simulink model "Admittace_Control"  (R2020a)
settings: Solver=FixedStepAuto  StartTime=0.0  StopTime=2  FixedStep=0.001  RelTol=1e-3  EnableMultiTasking=on
undefined symbols (not defined in the file or in its folder): X, Y, Z
libraries: sm_lib x79, nesl_utility x41, roblocks x8
(part 1 of 3)
settings Model: Creator=Administrator  LastModifiedBy=hemingshan
settings DataIOCC: ReturnWorkspaceOutputs=off
settings OptimizationCC: LifeSpan=inf
settings DebuggingCC: SFUnexpectedBacktrackingDiag=warning  SFNoUnconditionalDefaultTransitionDiag=warning  ArithmeticOperatorsInVariantConditions=warning
settings SFSimCC: SimUseLocalCustomCode=off  CustomCodeUndefinedFunction=UseInterfaceOnly
settings RTWCC: RTWUseLocalCustomCode=off
settings CodeAppCC: StateflowObjectComments=on
settings GRTTargetCC: TargetLangStandard=C89/C90 (ANSI)
settings ConfigComp: CovMetricSettings=dw  CovHtmlReporting=on  CovSaveCumulativeToWorkspaceVar=on  CovSaveSingleToWorkspaceVar=on  CovExternalEMLEnable=off
settings SimscapeCC: SimscapeNormalizeSystem=off

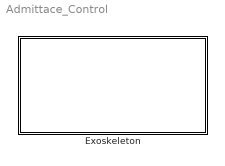
== system Admittace_Control ==
  Exoskeleton : Subsystem
      mask Display: disp('Admittance Control');

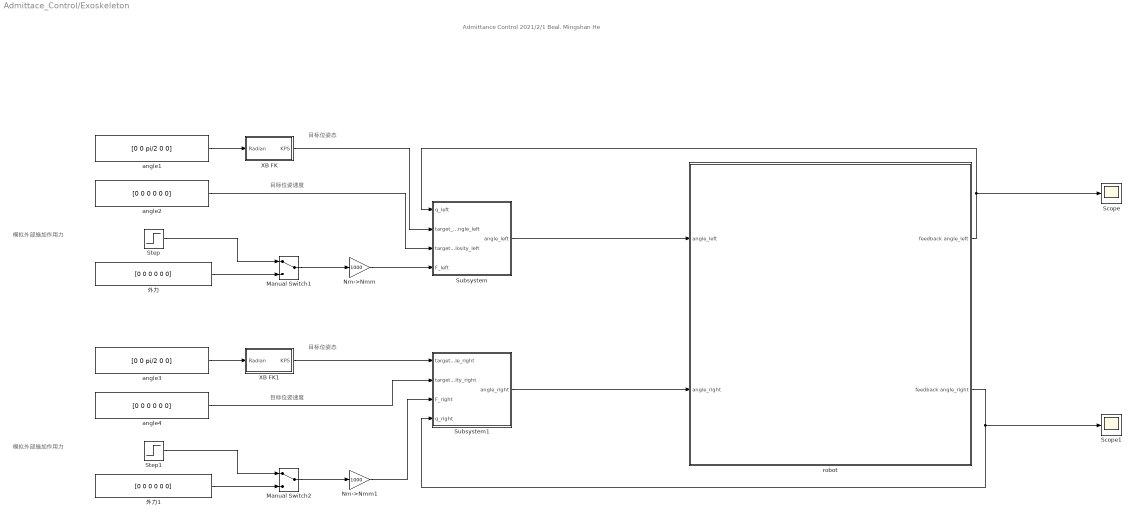
== system Admittace_Control/Exoskeleton ==
  note: Admittance Control
      | 2021/2/1
      | Beal. Mingshan He
  note: 目标位姿速度
  note: 目标位姿态
  note: 模拟外部施加作用力
  note: 模拟外部施加作用力
  note: 目标位姿速度
  note: 目标位姿态
  Manual Switch1 : ManualSwitch
  Manual Switch2 : ManualSwitch
  Nm->Nmm : Gain  Gain=1000
  Nm->Nmm1 : Gain  Gain=1000
  Scope : Scope
  Scope1 : Scope
  Step : Step  Before=[0.1 0 10 0 0 0]  After=[0 0 0 0 0 0]  SampleTime=0
  Step1 : Step  Before=[0.1 0 10 0 0 0]  After=[0 0 0 0 0 0]  SampleTime=0
  Subsystem : Subsystem
  Subsystem1 : Subsystem
  XB FK : Subsystem
  XB FK1 : Subsystem
  angle1 : Constant  Value=[0 0 pi/2 0 0]
  angle2 : Constant  Value=[0 0 0 0 0 0]
  angle3 : Constant  Value=[0 0 pi/2 0 0]
  angle4 : Constant  Value=[0 0 0 0 0 0]
  robot : Subsystem
  外力 : Constant  Value=[0 0 0 0 0 0]
  外力1 : Constant  Value=[0 0 0 0 0 0]
  wires:
  Step/1 -> Manual Switch1/1
  angle1/1 -> XB FK/1(Radian)
  Manual Switch1/1 -> Nm->Nmm/1
  外力/1 -> Manual Switch1/2
  robot/1(feedback angle_left) -> Subsystem/1(q_left), Scope/1
  XB FK/1(KPS) -> Subsystem/2(target_angle_left)
  angle2/1 -> Subsystem/3(target_velosity_left)
  Nm->Nmm/1 -> Subsystem/4(F_left)
  Subsystem/1(angle_left) -> robot/1(angle_left)
  Subsystem1/1(angle_right) -> robot/2(angle_right)
  robot/2(feedback angle_right) -> Subsystem1/4(q_right), Scope1/1
  Nm->Nmm1/1 -> Subsystem1/3(F_right)
  Manual Switch2/1 -> Nm->Nmm1/1
  Step1/1 -> Manual Switch2/1
  外力1/1 -> Manual Switch2/2
  angle3/1 -> XB FK1/1(Radian)
  XB FK1/1(KPS) -> Subsystem1/1(target_angle_right)
  angle4/1 -> Subsystem1/2(target_velosity_right)

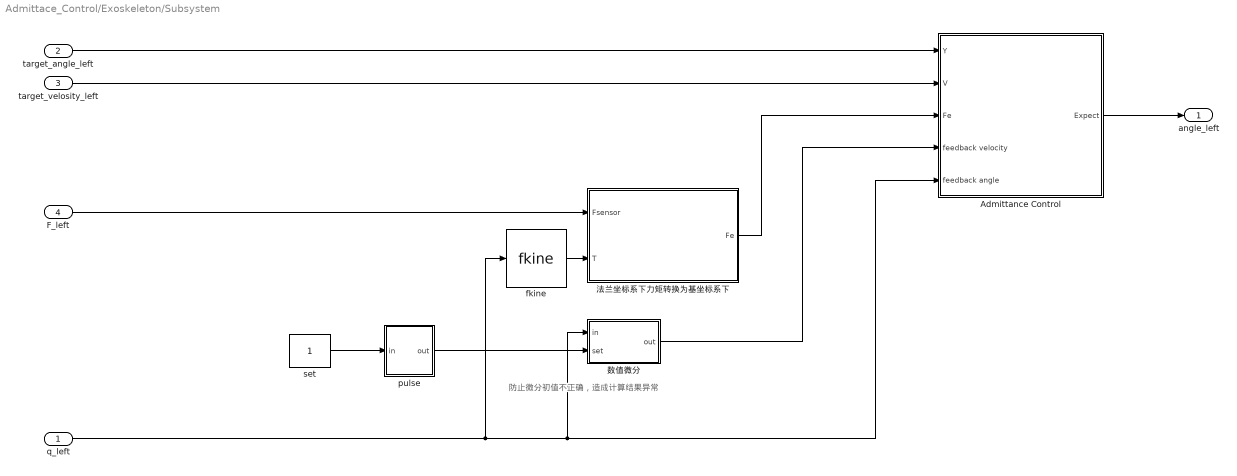
== system Admittace_Control/Exoskeleton/Subsystem ==
  note: 防止微分初值不正确，造成计算结果异常
  q_left : Inport
  target_angle_left : Inport  Port=2
  target_velosity_left : Inport  Port=3
  F_left : Inport  Port=4
  Admittance Control : Subsystem  mask{m_M=[1 1 1 1 1 1], m_B=[100 100 100 200 200 200], m_K=[250 250 250 1000 1000 1000]}
      mask prompts: m_M "M"; m_B "B"; m_K "K"
  fkine : roblocks/Arm/fkine  robot=robot
  pulse : MATLAB Function  TreatAsAtomicUnit=on
  set : Constant
  数值微分 : MATLAB Function  TreatAsAtomicUnit=on
  法兰坐标系下力矩转换为基坐标系下 : MATLAB Function  TreatAsAtomicUnit=on
  angle_left : Outport
  wires:
  fkine/1 -> 法兰坐标系下力矩转换为基坐标系下/2(T)
  法兰坐标系下力矩转换为基坐标系下/1(Fe) -> Admittance Control/3(Fe)
  pulse/1(out) -> 数值微分/2(set)
  target_angle_left/1 -> Admittance Control/1(Y)
  数值微分/1(out) -> Admittance Control/4(feedback velocity)
  F_left/1 -> 法兰坐标系下力矩转换为基坐标系下/1(Fsensor)
  set/1 -> pulse/1(in)
  q_left/1 -> Admittance Control/5(feedback angle), 数值微分/1(in), fkine/1
  target_velosity_left/1 -> Admittance Control/2(V)
  Admittance Control/1(Expect) -> angle_left/1

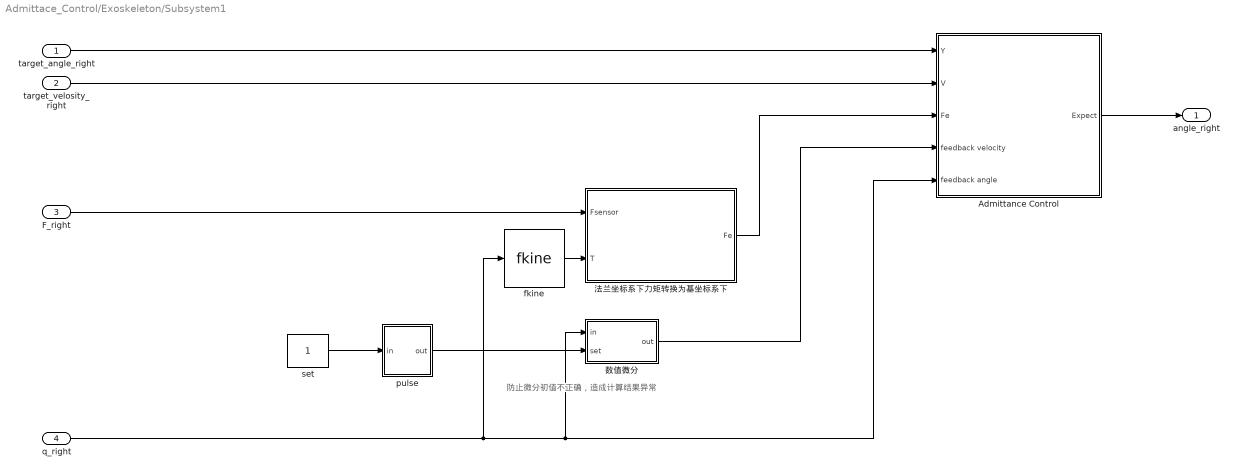
== system Admittace_Control/Exoskeleton/Subsystem1 ==
  note: 防止微分初值不正确，造成计算结果异常
  target_angle_right : Inport
  target_velosity_right : Inport  Port=2
  F_right : Inport  Port=3
  q_right : Inport  Port=4
  Admittance Control : Subsystem  mask{m_M=[1 1 1 1 1 1], m_B=[100 100 100 200 200 200], m_K=[250 250 250 1000 1000 1000]}
      mask prompts: m_M "M"; m_B "B"; m_K "K"
  fkine : roblocks/Arm/fkine  robot=robot
  pulse : MATLAB Function  TreatAsAtomicUnit=on
  set : Constant
  数值微分 : MATLAB Function  TreatAsAtomicUnit=on
  法兰坐标系下力矩转换为基坐标系下 : MATLAB Function  TreatAsAtomicUnit=on
  angle_right : Outport
  wires:
  fkine/1 -> 法兰坐标系下力矩转换为基坐标系下/2(T)
  法兰坐标系下力矩转换为基坐标系下/1(Fe) -> Admittance Control/3(Fe)
  pulse/1(out) -> 数值微分/2(set)
  target_angle_right/1 -> Admittance Control/1(Y)
  数值微分/1(out) -> Admittance Control/4(feedback velocity)
  F_right/1 -> 法兰坐标系下力矩转换为基坐标系下/1(Fsensor)
  set/1 -> pulse/1(in)
  q_right/1 -> Admittance Control/5(feedback angle), 数值微分/1(in), fkine/1
  target_velosity_right/1 -> Admittance Control/2(V)
  Admittance Control/1(Expect) -> angle_right/1

== system Admittace_Control/Exoskeleton/XB FK ==
  Radian : Inport
  DH-CC1 : MATLAB Function  TreatAsAtomicUnit=on
  fkine1 : roblocks/Arm/fkine  robot=robot
  KPS : Outport  VectorParamsAs1DForOutWhenUnconnected=off
  wires:
  fkine1/1 -> DH-CC1/1(KPS44)
  DH-CC1/1(KPS6) -> KPS/1
  Radian/1 -> fkine1/1

== system Admittace_Control/Exoskeleton/XB FK1 ==
  Radian : Inport
  DH-CC1 : MATLAB Function  TreatAsAtomicUnit=on
  fkine1 : roblocks/Arm/fkine  robot=robot
  KPS : Outport  VectorParamsAs1DForOutWhenUnconnected=off
  wires:
  fkine1/1 -> DH-CC1/1(KPS44)
  DH-CC1/1(KPS6) -> KPS/1
  Radian/1 -> fkine1/1

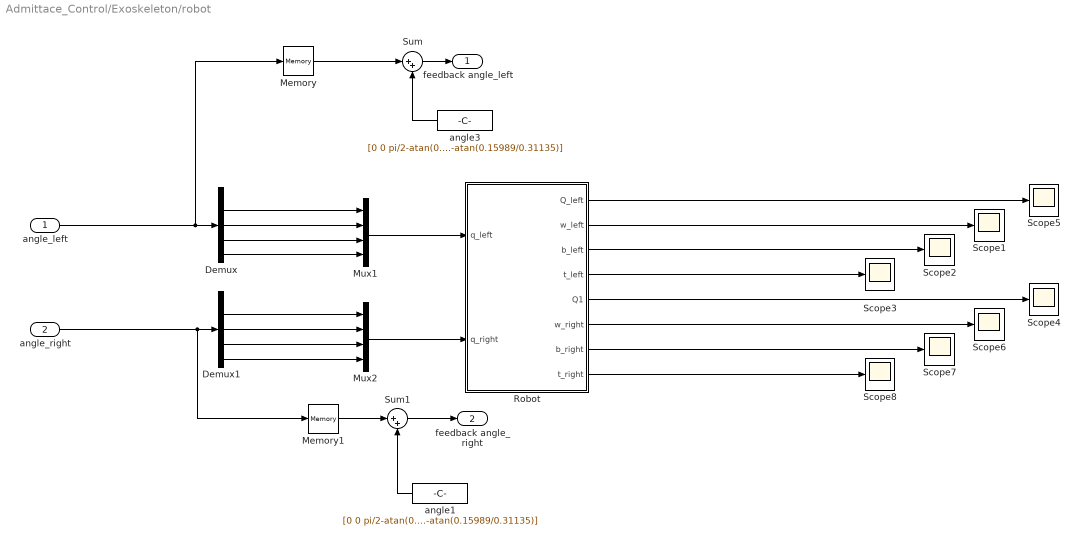
== system Admittace_Control/Exoskeleton/robot ==
  angle_left : Inport
  angle_right : Inport  Port=2
  Demux : Demux  Outputs=5
  Demux1 : Demux  Outputs=5
  Memory : Memory  InitialCondition=[0 0 0 0 0]
  Memory1 : Memory  InitialCondition=[0 0 0 0 0]
  Mux1 : Mux
  Mux2 : Mux
  Robot : Subsystem
  Scope{1..8} (8 alike) : Scope
  Sum : Sum  Inputs=|++
  Sum1 : Sum  Inputs=|++
  angle1 : Constant  Value=[0 0 pi/2-atan(0.23966/0.28189) pi/2-atan(0.23966/0.28189)+atan(0.15989/0.31135) -atan(0.15989/0.31135)]
  angle3 : Constant  Value=[0 0 pi/2-atan(0.23966/0.28189) pi/2-atan(0.23966/0.28189)+atan(0.15989/0.31135) -atan(0.15989/0.31135)]
  feedback angle_left : Outport  VectorParamsAs1DForOutWhenUnconnected=off
  feedback angle_right : Outport  Port=2  VectorParamsAs1DForOutWhenUnconnected=off
  wires:
  Robot/1(Q_left) -> Scope5/1
  Robot/2(w_left) -> Scope1/1
  Robot/3(b_left) -> Scope2/1
  Robot/4(t_left) -> Scope3/1
  angle_left/1 -> Memory/1, Demux/1
  Mux1/1 -> Robot/1(q_left)
  Demux/2 -> Mux1/1
  Demux/3 -> Mux1/2
  Demux/4 -> Mux1/3
  Demux/5 -> Mux1/4
  Robot/5(Q1) -> Scope4/1
  Robot/6(w_right) -> Scope6/1
  Robot/7(b_right) -> Scope7/1
  Robot/8(t_right) -> Scope8/1
  angle_right/1 -> Memory1/1, Demux1/1
  Demux1/5 -> Mux2/4
  Demux1/4 -> Mux2/3
  Demux1/3 -> Mux2/2
  Demux1/2 -> Mux2/1
  Mux2/1 -> Robot/2(q_right)
  angle3/1 -> Sum/2
  Memory/1 -> Sum/1
  Sum/1 -> feedback angle_left/1
  Memory1/1 -> Sum1/1
  Sum1/1 -> feedback angle_right/1
  angle1/1 -> Sum1/2

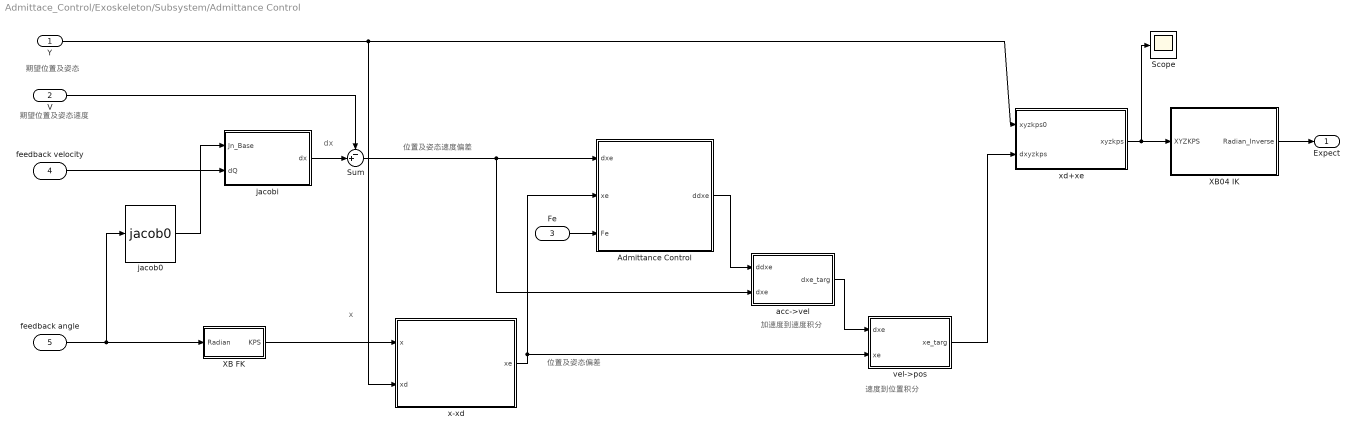
== system Admittace_Control/Exoskeleton/Subsystem/Admittance Control ==
  note: 加速度到速度积分
  note: 期望位置及姿态速度
  note: dx
  note: x
  note: 期望位置及姿态
  note: 位置及姿态偏差
  note: 位置及姿态速度偏差
  note: 速度到位置积分
  Y : Inport
  V : Inport  Port=2
  Fe : Inport  Port=3
  feedback velocity : Inport  Port=4
  feedback angle : Inport  Port=5
  Admittance Control : MATLAB Function  TreatAsAtomicUnit=on
  Scope : Scope
  Sum : Sum  Inputs=-+|
  XB FK : Subsystem
  XB04 IK : Subsystem
  acc->vel : MATLAB Function  TreatAsAtomicUnit=on
  "jacob0 " : roblocks/Arm/jacob0   robot=robot
  jacobi : MATLAB Function  TreatAsAtomicUnit=on
  vel->pos : MATLAB Function  TreatAsAtomicUnit=on
  x-xd : MATLAB Function  TreatAsAtomicUnit=on
  xd+xe : MATLAB Function  TreatAsAtomicUnit=on
  Expect : Outport  VectorParamsAs1DForOutWhenUnconnected=off
  wires:
  Fe/1 -> Admittance Control/3(Fe)
  Admittance Control/1(ddxe) -> acc->vel/1(ddxe)
  Y/1 -> xd+xe/1(xyzkps0), x-xd/2(xd)
  XB FK/1(KPS) -> x-xd/1(x)
  x-xd/1(xe) -> Admittance Control/2(xe), vel->pos/2(xe)
  vel->pos/1(xe_targ) -> xd+xe/2(dxyzkps)
  jacobi/1(dx) -> Sum/2
  Sum/1 -> acc->vel/2(dxe), Admittance Control/1(dxe)
  acc->vel/1(dxe_targ) -> vel->pos/1(dxe)
  xd+xe/1(xyzkps) -> Scope/1, XB04 IK/1(XYZKPS)
  V/1 -> Sum/1
  feedback velocity/1 -> jacobi/2(dQ)
  XB04 IK/1(Radian_Inverse) -> Expect/1
  feedback angle/1 -> "jacob0 "/1, XB FK/1(Radian)
  "jacob0 "/1 -> jacobi/1(Jn_Base)

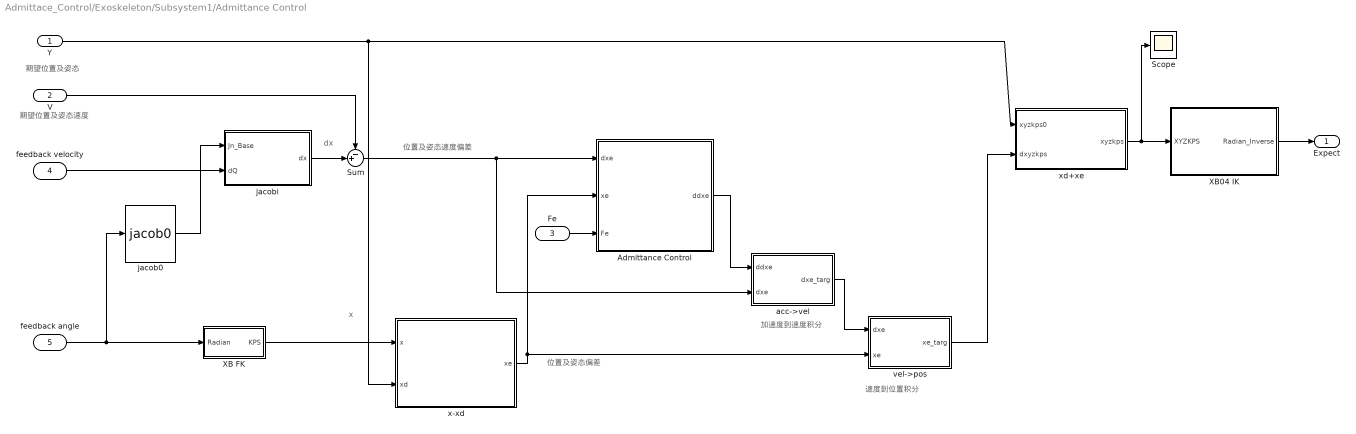
== system Admittace_Control/Exoskeleton/Subsystem1/Admittance Control ==
  note: 加速度到速度积分
  note: 期望位置及姿态速度
  note: dx
  note: x
  note: 期望位置及姿态
  note: 位置及姿态偏差
  note: 位置及姿态速度偏差
  note: 速度到位置积分
  Y : Inport
  V : Inport  Port=2
  Fe : Inport  Port=3
  feedback velocity : Inport  Port=4
  feedback angle : Inport  Port=5
  Admittance Control : MATLAB Function  TreatAsAtomicUnit=on
  Scope : Scope
  Sum : Sum  Inputs=-+|
  XB FK : Subsystem
  XB04 IK : Subsystem
  acc->vel : MATLAB Function  TreatAsAtomicUnit=on
  "jacob0 " : roblocks/Arm/jacob0   robot=robot
  jacobi : MATLAB Function  TreatAsAtomicUnit=on
  vel->pos : MATLAB Function  TreatAsAtomicUnit=on
  x-xd : MATLAB Function  TreatAsAtomicUnit=on
  xd+xe : MATLAB Function  TreatAsAtomicUnit=on
  Expect : Outport  VectorParamsAs1DForOutWhenUnconnected=off
  wires:
  Fe/1 -> Admittance Control/3(Fe)
  Admittance Control/1(ddxe) -> acc->vel/1(ddxe)
  Y/1 -> xd+xe/1(xyzkps0), x-xd/2(xd)
  XB FK/1(KPS) -> x-xd/1(x)
  x-xd/1(xe) -> Admittance Control/2(xe), vel->pos/2(xe)
  vel->pos/1(xe_targ) -> xd+xe/2(dxyzkps)
  jacobi/1(dx) -> Sum/2
  Sum/1 -> acc->vel/2(dxe), Admittance Control/1(dxe)
  acc->vel/1(dxe_targ) -> vel->pos/1(dxe)
  xd+xe/1(xyzkps) -> Scope/1, XB04 IK/1(XYZKPS)
  V/1 -> Sum/1
  feedback velocity/1 -> jacobi/2(dQ)
  XB04 IK/1(Radian_Inverse) -> Expect/1
  feedback angle/1 -> "jacob0 "/1, XB FK/1(Radian)
  "jacob0 "/1 -> jacobi/1(Jn_Base)

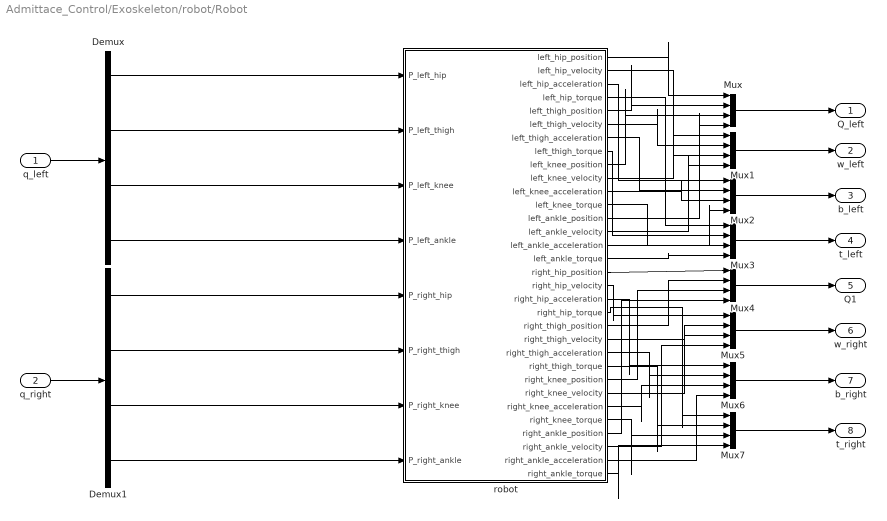
== system Admittace_Control/Exoskeleton/robot/Robot ==
  q_left : Inport
  q_right : Inport  Port=2
  Demux : Demux
  Demux1 : Demux
  Mux{,1..7} (8 alike) : Mux
  robot : Subsystem
  Q_left : Outport  VectorParamsAs1DForOutWhenUnconnected=off
  w_left : Outport  Port=2  VectorParamsAs1DForOutWhenUnconnected=off
  b_left : Outport  Port=3  VectorParamsAs1DForOutWhenUnconnected=off
  t_left : Outport  Port=4  VectorParamsAs1DForOutWhenUnconnected=off
  Q1 : Outport  Port=5  VectorParamsAs1DForOutWhenUnconnected=off
  w_right : Outport  Port=6  VectorParamsAs1DForOutWhenUnconnected=off
  b_right : Outport  Port=7  VectorParamsAs1DForOutWhenUnconnected=off
  t_right : Outport  Port=8  VectorParamsAs1DForOutWhenUnconnected=off
  wires:
  q_left/1 -> Demux/1
  Mux/1 -> Q_left/1
  Mux1/1 -> w_left/1
  Mux2/1 -> b_left/1
  Mux3/1 -> t_left/1
  Demux/1 -> robot/1(P_left_hip)
  Demux/2 -> robot/2(P_left_thigh)
  Demux/3 -> robot/3(P_left_knee)
  Demux/4 -> robot/4(P_left_ankle)
  robot/1(left_hip_position) -> Mux/1
  robot/5(left_thigh_position) -> Mux/2
  robot/9(left_knee_position) -> Mux/3
  robot/13(left_ankle_position) -> Mux/4
  robot/2(left_hip_velocity) -> Mux1/1
  robot/6(left_thigh_velocity) -> Mux1/2
  robot/10(left_knee_velocity) -> Mux1/3
  robot/14(left_ankle_velocity) -> Mux1/4
  robot/16(left_ankle_torque) -> Mux3/4
  robot/12(left_knee_torque) -> Mux3/3
  robot/8(left_thigh_torque) -> Mux3/2
  robot/4(left_hip_torque) -> Mux3/1
  robot/15(left_ankle_acceleration) -> Mux2/4
  robot/11(left_knee_acceleration) -> Mux2/3
  robot/7(left_thigh_acceleration) -> Mux2/2
  robot/3(left_hip_acceleration) -> Mux2/1
  q_right/1 -> Demux1/1
  Demux1/1 -> robot/5(P_right_hip)
  Demux1/2 -> robot/6(P_right_thigh)
  Demux1/3 -> robot/7(P_right_knee)
  Demux1/4 -> robot/8(P_right_ankle)
  Mux4/1 -> Q1/1
  robot/17(right_hip_position) -> Mux4/1
  robot/21(right_thigh_position) -> Mux4/2
  robot/25(right_knee_position) -> Mux4/3
  robot/29(right_ankle_position) -> Mux4/4
  robot/18(right_hip_velocity) -> Mux5/1
  robot/22(right_thigh_velocity) -> Mux5/2
  robot/26(right_knee_velocity) -> Mux5/3
  robot/30(right_ankle_velocity) -> Mux5/4
  robot/19(right_hip_acceleration) -> Mux6/1
  robot/23(right_thigh_acceleration) -> Mux6/2
  robot/27(right_knee_acceleration) -> Mux6/3
  robot/31(right_ankle_acceleration) -> Mux6/4
  robot/20(right_hip_torque) -> Mux7/1
  robot/24(right_thigh_torque) -> Mux7/2
  robot/28(right_knee_torque) -> Mux7/3
  robot/32(right_ankle_torque) -> Mux7/4
  Mux5/1 -> w_right/1
  Mux6/1 -> b_right/1
  Mux7/1 -> t_right/1

== system Admittace_Control/Exoskeleton/Subsystem/Admittance Control/XB FK ==
  Radian : Inport
  DH-CC1 : MATLAB Function  TreatAsAtomicUnit=on
  fkine1 : roblocks/Arm/fkine  robot=robot
  KPS : Outport  VectorParamsAs1DForOutWhenUnconnected=off
  wires:
  fkine1/1 -> DH-CC1/1(KPS44)
  DH-CC1/1(KPS6) -> KPS/1
  Radian/1 -> fkine1/1

== system Admittace_Control/Exoskeleton/Subsystem/Admittance Control/XB04 IK ==
  XYZKPS : Inport
  Constant : Constant  Value=[0 0 pi/2-atan(0.23966/0.28189) pi/2-atan(0.23966/0.28189)+atan(0.15989/0.31135) -atan(0.15989/0.31135)]
  DH-IK-CC : MATLAB Function  TreatAsAtomicUnit=on
  Display : Display
  MATLAB Function : MATLAB Function  TreatAsAtomicUnit=on
  Sum : Sum  Inputs=|+-
  Radian_Inverse : Outport  VectorParamsAs1DForOutWhenUnconnected=off
  wires:
  XYZKPS/1 -> DH-IK-CC/1(KPS6)
  DH-IK-CC/1(KPS44) -> MATLAB Function/1(T), Display/1
  MATLAB Function/1(q) -> Sum/1
  Sum/1 -> Radian_Inverse/1
  Constant/1 -> Sum/2

== system Admittace_Control/Exoskeleton/Subsystem1/Admittance Control/XB FK ==
  Radian : Inport
  DH-CC1 : MATLAB Function  TreatAsAtomicUnit=on
  fkine1 : roblocks/Arm/fkine  robot=robot
  KPS : Outport  VectorParamsAs1DForOutWhenUnconnected=off
  wires:
  fkine1/1 -> DH-CC1/1(KPS44)
  DH-CC1/1(KPS6) -> KPS/1
  Radian/1 -> fkine1/1

== system Admittace_Control/Exoskeleton/Subsystem1/Admittance Control/XB04 IK ==
  XYZKPS : Inport
  Constant : Constant  Value=[0 0 pi/2-atan(0.23966/0.28189) pi/2-atan(0.23966/0.28189)+atan(0.15989/0.31135) -atan(0.15989/0.31135)]
  DH-IK-CC : MATLAB Function  TreatAsAtomicUnit=on
  Display : Display
  MATLAB Function : MATLAB Function  TreatAsAtomicUnit=on
  Sum : Sum  Inputs=|+-
  Radian_Inverse : Outport  VectorParamsAs1DForOutWhenUnconnected=off
  wires:
  XYZKPS/1 -> DH-IK-CC/1(KPS6)
  DH-IK-CC/1(KPS44) -> MATLAB Function/1(T), Display/1
  MATLAB Function/1(q) -> Sum/1
  Sum/1 -> Radian_Inverse/1
  Constant/1 -> Sum/2

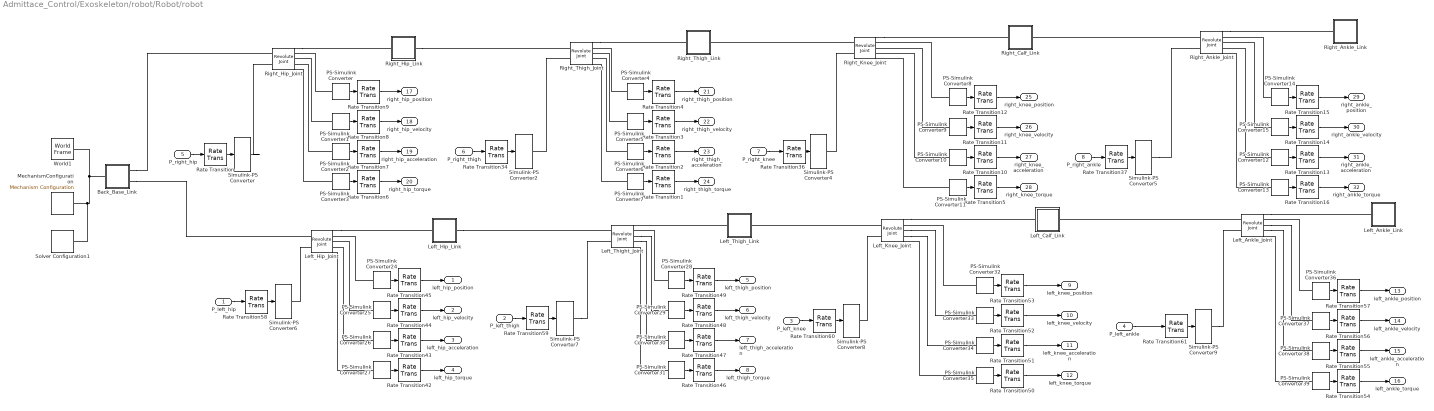
== system Admittace_Control/Exoskeleton/robot/Robot/robot ==
  P_left_hip : Inport
  P_left_thigh : Inport  Port=2
  P_left_knee : Inport  Port=3
  P_left_ankle : Inport  Port=4
  P_right_hip : Inport  Port=5
  P_right_thigh : Inport  Port=6
  P_right_knee : Inport  Port=7
  P_right_ankle : Inport  Port=8
  Back_Base_Link : Subsystem
  Left_Ankle_Joint : sm_lib/Joints/Revolute Joint  JointMode=Normal  SenseConstraintForce=off  SenseConstraintForceX=off  SenseConstraintForceY=off  SenseConstraintForceZ=off  SenseConstraintTorque=off  SenseConstraintTorqueX=off  SenseConstraintTorqueY=off  SenseConstraintTorqueZ=off  SenseTotalForce=off  SenseTotalForceX=off  SenseTotalForceY=off  SenseTotalForceZ=off  SenseTotalTorque=off  SenseTotalTorqueX=off  SenseTotalTorqueY=off  SenseTotalTorqueZ=off  CompositeWrenchDir=FollowerOnBase  CompositeWrenchFrame=BaseFrame  EquilibriumPosition=0  EquilibriumPositionUnits=deg  SpringStiffness=0  SpringStiffnessUnits=N*m/deg  DampingCoefficient=0  DampingCoefficientUnits=m^2*kg/s/rad  TorqueActuationMode=ComputedTorque  MotionActuationMode=InputMotion  SensePosition=on  SenseVelocity=on  SenseAcceleration=on  SenseTorqueForce=on  SenseLowerLimitTorqueForce=off  SenseUpperLimitTorqueForce=off  LowerLimitSpecify=off  LowerLimitBound=0  LowerLimitBoundUnits=rad  LowerLimitStiffness=1e4  LowerLimitStiffnessUnits=N*m/deg  LowerLimitDamping=10  LowerLimitDampingUnits=N*m/(deg/s)  LowerLimitTransitionRegionWidth=0.1  LowerLimitTransitionRegionWidthUnits=deg  UpperLimitSpecify=off  UpperLimitBound=0  UpperLimitBoundUnits=rad  UpperLimitStiffness=1e4  UpperLimitStiffnessUnits=N*m/deg  UpperLimitDamping=10  UpperLimitDampingUnits=N*m/(deg/s)  UpperLimitTransitionRegionWidth=0.1  UpperLimitTransitionRegionWidthUnits=deg  PositionTargetSpecify=off  PositionTargetPriority=High  PositionTargetValue=0  PositionTargetValueUnits=deg  VelocityTargetSpecify=off  VelocityTargetPriority=High  VelocityTargetValue=0  VelocityTargetValueUnits=deg/s
  Left_Ankle_Link : Subsystem
  Left_Calf_Link : Subsystem
  Left_Hip_Joint : sm_lib/Joints/Revolute Joint  JointMode=Normal  SenseConstraintForce=off  SenseConstraintForceX=off  SenseConstraintForceY=off  SenseConstraintForceZ=off  SenseConstraintTorque=off  SenseConstraintTorqueX=off  SenseConstraintTorqueY=off  SenseConstraintTorqueZ=off  SenseTotalForce=off  SenseTotalForceX=off  SenseTotalForceY=off  SenseTotalForceZ=off  SenseTotalTorque=off  SenseTotalTorqueX=off  SenseTotalTorqueY=off  SenseTotalTorqueZ=off  CompositeWrenchDir=FollowerOnBase  CompositeWrenchFrame=BaseFrame  EquilibriumPosition=0  EquilibriumPositionUnits=deg  SpringStiffness=0  SpringStiffnessUnits=N*m/deg  DampingCoefficient=0  DampingCoefficientUnits=m^2*kg/s/rad  TorqueActuationMode=ComputedTorque  MotionActuationMode=InputMotion  SensePosition=on  SenseVelocity=on  SenseAcceleration=on  SenseTorqueForce=on  SenseLowerLimitTorqueForce=off  SenseUpperLimitTorqueForce=off  LowerLimitSpecify=off  LowerLimitBound=0  LowerLimitBoundUnits=rad  LowerLimitStiffness=1e4  LowerLimitStiffnessUnits=N*m/deg  LowerLimitDamping=10  LowerLimitDampingUnits=N*m/(deg/s)  LowerLimitTransitionRegionWidth=0.1  LowerLimitTransitionRegionWidthUnits=deg  UpperLimitSpecify=off  UpperLimitBound=0  UpperLimitBoundUnits=rad  UpperLimitStiffness=1e4  UpperLimitStiffnessUnits=N*m/deg  UpperLimitDamping=10  UpperLimitDampingUnits=N*m/(deg/s)  UpperLimitTransitionRegionWidth=0.1  UpperLimitTransitionRegionWidthUnits=deg  PositionTargetSpecify=off  PositionTargetPriority=High  PositionTargetValue=0  PositionTargetValueUnits=deg  VelocityTargetSpecify=off  VelocityTargetPriority=High  VelocityTargetValue=0  VelocityTargetValueUnits=deg/s
  Left_Hip_Link : Subsystem
  Left_Knee_Joint : sm_lib/Joints/Revolute Joint  JointMode=Normal  SenseConstraintForce=off  SenseConstraintForceX=off  SenseConstraintForceY=off  SenseConstraintForceZ=off  SenseConstraintTorque=off  SenseConstraintTorqueX=off  SenseConstraintTorqueY=off  SenseConstraintTorqueZ=off  SenseTotalForce=off  SenseTotalForceX=off  SenseTotalForceY=off  SenseTotalForceZ=off  SenseTotalTorque=off  SenseTotalTorqueX=off  SenseTotalTorqueY=off  SenseTotalTorqueZ=off  CompositeWrenchDir=FollowerOnBase  CompositeWrenchFrame=BaseFrame  EquilibriumPosition=0  EquilibriumPositionUnits=deg  SpringStiffness=0  SpringStiffnessUnits=N*m/deg  DampingCoefficient=0  DampingCoefficientUnits=m^2*kg/s/rad  TorqueActuationMode=ComputedTorque  MotionActuationMode=InputMotion  SensePosition=on  SenseVelocity=on  SenseAcceleration=on  SenseTorqueForce=on  SenseLowerLimitTorqueForce=off  SenseUpperLimitTorqueForce=off  LowerLimitSpecify=off  LowerLimitBound=0  LowerLimitBoundUnits=rad  LowerLimitStiffness=1e4  LowerLimitStiffnessUnits=N*m/deg  LowerLimitDamping=10  LowerLimitDampingUnits=N*m/(deg/s)  LowerLimitTransitionRegionWidth=0.1  LowerLimitTransitionRegionWidthUnits=deg  UpperLimitSpecify=off  UpperLimitBound=0  UpperLimitBoundUnits=rad  UpperLimitStiffness=1e4  UpperLimitStiffnessUnits=N*m/deg  UpperLimitDamping=10  UpperLimitDampingUnits=N*m/(deg/s)  UpperLimitTransitionRegionWidth=0.1  UpperLimitTransitionRegionWidthUnits=deg  PositionTargetSpecify=off  PositionTargetPriority=High  PositionTargetValue=0  PositionTargetValueUnits=deg  VelocityTargetSpecify=off  VelocityTargetPriority=High  VelocityTargetValue=0  VelocityTargetValueUnits=deg/s
  Left_Thigh_Link : Subsystem
  Left_Thight_Joint : sm_lib/Joints/Revolute Joint  JointMode=Normal  SenseConstraintForce=off  SenseConstraintForceX=off  SenseConstraintForceY=off  SenseConstraintForceZ=off  SenseConstraintTorque=off  SenseConstraintTorqueX=off  SenseConstraintTorqueY=off  SenseConstraintTorqueZ=off  SenseTotalForce=off  SenseTotalForceX=off  SenseTotalForceY=off  SenseTotalForceZ=off  SenseTotalTorque=off  SenseTotalTorqueX=off  SenseTotalTorqueY=off  SenseTotalTorqueZ=off  CompositeWrenchDir=FollowerOnBase  CompositeWrenchFrame=BaseFrame  EquilibriumPosition=0  EquilibriumPositionUnits=deg  SpringStiffness=0  SpringStiffnessUnits=N*m/deg  DampingCoefficient=0  DampingCoefficientUnits=m^2*kg/s/rad  TorqueActuationMode=ComputedTorque  MotionActuationMode=InputMotion  SensePosition=on  SenseVelocity=on  SenseAcceleration=on  SenseTorqueForce=on  SenseLowerLimitTorqueForce=off  SenseUpperLimitTorqueForce=off  LowerLimitSpecify=off  LowerLimitBound=0  LowerLimitBoundUnits=rad  LowerLimitStiffness=1e4  LowerLimitStiffnessUnits=N*m/deg  LowerLimitDamping=10  LowerLimitDampingUnits=N*m/(deg/s)  LowerLimitTransitionRegionWidth=0.1  LowerLimitTransitionRegionWidthUnits=deg  UpperLimitSpecify=off  UpperLimitBound=0  UpperLimitBoundUnits=rad  UpperLimitStiffness=1e4  UpperLimitStiffnessUnits=N*m/deg  UpperLimitDamping=10  UpperLimitDampingUnits=N*m/(deg/s)  UpperLimitTransitionRegionWidth=0.1  UpperLimitTransitionRegionWidthUnits=deg  PositionTargetSpecify=off  PositionTargetPriority=High  PositionTargetValue=0  PositionTargetValueUnits=deg  VelocityTargetSpecify=off  VelocityTargetPriority=High  VelocityTargetValue=0  VelocityTargetValueUnits=deg/s
  MechanismConfiguration : sm_lib/Utilities/Mechanism Configuration  UniformGravity=Constant  GravityVector=[0 0 -9.80665]  GravityUnits=m/s^2  LinearizationDelta=0.001
  PS-Simulink Converter{,4,8,14,24,28,32,36} (8 alike) : nesl_utility/PS-Simulink Converter  PhysicalDomain=network_engine_domain  SubClassName=ps_output  LeftPortType=input  RightPortType=output  PseudoPeriodic=off  Frequencies=[]  Unit=rad  AffineConversion=off
  PS-Simulink Converter{1,5,9,15,25,29,33,37} (8 alike) : nesl_utility/PS-Simulink Converter  PhysicalDomain=network_engine_domain  SubClassName=ps_output  LeftPortType=input  RightPortType=output  PseudoPeriodic=off  Frequencies=[]  Unit=rad/s  AffineConversion=off
  PS-Simulink Converter{2,6,10,12,26,30,34,38} (8 alike) : nesl_utility/PS-Simulink Converter  PhysicalDomain=network_engine_domain  SubClassName=ps_output  LeftPortType=input  RightPortType=output  PseudoPeriodic=off  Frequencies=[]  Unit=1  AffineConversion=off
  PS-Simulink Converter{3,7,11,13,27,31,35,39} (8 alike) : nesl_utility/PS-Simulink Converter  PhysicalDomain=network_engine_domain  SubClassName=ps_output  LeftPortType=input  RightPortType=output  PseudoPeriodic=off  Frequencies=[]  Unit=N*m  AffineConversion=off
  Rate Transition{,1..16,34,36..37,42..61} (40 alike) : RateTransition
  Right_Ankle_Joint : sm_lib/Joints/Revolute Joint  JointMode=Normal  SenseConstraintForce=off  SenseConstraintForceX=off  SenseConstraintForceY=off  SenseConstraintForceZ=off  SenseConstraintTorque=off  SenseConstraintTorqueX=off  SenseConstraintTorqueY=off  SenseConstraintTorqueZ=off  SenseTotalForce=off  SenseTotalForceX=off  SenseTotalForceY=off  SenseTotalForceZ=off  SenseTotalTorque=off  SenseTotalTorqueX=off  SenseTotalTorqueY=off  SenseTotalTorqueZ=off  CompositeWrenchDir=FollowerOnBase  CompositeWrenchFrame=BaseFrame  EquilibriumPosition=0  EquilibriumPositionUnits=deg  SpringStiffness=0  SpringStiffnessUnits=N*m/deg  DampingCoefficient=0  DampingCoefficientUnits=m^2*kg/s/rad  TorqueActuationMode=ComputedTorque  MotionActuationMode=InputMotion  SensePosition=on  SenseVelocity=on  SenseAcceleration=on  SenseTorqueForce=on  SenseLowerLimitTorqueForce=off  SenseUpperLimitTorqueForce=off  LowerLimitSpecify=off  LowerLimitBound=0  LowerLimitBoundUnits=rad  LowerLimitStiffness=1e4  LowerLimitStiffnessUnits=N*m/deg  LowerLimitDamping=10  LowerLimitDampingUnits=N*m/(deg/s)  LowerLimitTransitionRegionWidth=0.1  LowerLimitTransitionRegionWidthUnits=deg  UpperLimitSpecify=off  UpperLimitBound=0  UpperLimitBoundUnits=rad  UpperLimitStiffness=1e4  UpperLimitStiffnessUnits=N*m/deg  UpperLimitDamping=10  UpperLimitDampingUnits=N*m/(deg/s)  UpperLimitTransitionRegionWidth=0.1  UpperLimitTransitionRegionWidthUnits=deg  PositionTargetSpecify=off  PositionTargetPriority=High  PositionTargetValue=0  PositionTargetValueUnits=deg  VelocityTargetSpecify=off  VelocityTargetPriority=High  VelocityTargetValue=0  VelocityTargetValueUnits=deg/s
  Right_Ankle_Link : Subsystem
  Right_Calf_Link : Subsystem
  Right_Hip_Joint : sm_lib/Joints/Revolute Joint  JointMode=Normal  SenseConstraintForce=off  SenseConstraintForceX=off  SenseConstraintForceY=off  SenseConstraintForceZ=off  SenseConstraintTorque=off  SenseConstraintTorqueX=off  SenseConstraintTorqueY=off  SenseConstraintTorqueZ=off  SenseTotalForce=off  SenseTotalForceX=off  SenseTotalForceY=off  SenseTotalForceZ=off  SenseTotalTorque=off  SenseTotalTorqueX=off  SenseTotalTorqueY=off  SenseTotalTorqueZ=off  CompositeWrenchDir=FollowerOnBase  CompositeWrenchFrame=BaseFrame  EquilibriumPosition=0  EquilibriumPositionUnits=deg  SpringStiffness=0  SpringStiffnessUnits=N*m/deg  DampingCoefficient=0  DampingCoefficientUnits=m^2*kg/s/rad  TorqueActuationMode=ComputedTorque  MotionActuationMode=InputMotion  SensePosition=on  SenseVelocity=on  SenseAcceleration=on  SenseTorqueForce=on  SenseLowerLimitTorqueForce=off  SenseUpperLimitTorqueForce=off  LowerLimitSpecify=off  LowerLimitBound=0  LowerLimitBoundUnits=rad  LowerLimitStiffness=1e4  LowerLimitStiffnessUnits=N*m/deg  LowerLimitDamping=10  LowerLimitDampingUnits=N*m/(deg/s)  LowerLimitTransitionRegionWidth=0.1  LowerLimitTransitionRegionWidthUnits=deg  UpperLimitSpecify=off  UpperLimitBound=0  UpperLimitBoundUnits=rad  UpperLimitStiffness=1e4  UpperLimitStiffnessUnits=N*m/deg  UpperLimitDamping=10  UpperLimitDampingUnits=N*m/(deg/s)  UpperLimitTransitionRegionWidth=0.1  UpperLimitTransitionRegionWidthUnits=deg  PositionTargetSpecify=off  PositionTargetPriority=High  PositionTargetValue=0  PositionTargetValueUnits=deg  VelocityTargetSpecify=off  VelocityTargetPriority=High  VelocityTargetValue=0  VelocityTargetValueUnits=deg/s
  Right_Hip_Link : Subsystem
  Right_Knee_Joint : sm_lib/Joints/Revolute Joint  JointMode=Normal  SenseConstraintForce=off  SenseConstraintForceX=off  SenseConstraintForceY=off  SenseConstraintForceZ=off  SenseConstraintTorque=off  SenseConstraintTorqueX=off  SenseConstraintTorqueY=off  SenseConstraintTorqueZ=off  SenseTotalForce=off  SenseTotalForceX=off  SenseTotalForceY=off  SenseTotalForceZ=off  SenseTotalTorque=off  SenseTotalTorqueX=off  SenseTotalTorqueY=off  SenseTotalTorqueZ=off  CompositeWrenchDir=FollowerOnBase  CompositeWrenchFrame=BaseFrame  EquilibriumPosition=0  EquilibriumPositionUnits=deg  SpringStiffness=0  SpringStiffnessUnits=N*m/deg  DampingCoefficient=0  DampingCoefficientUnits=m^2*kg/s/rad  TorqueActuationMode=ComputedTorque  MotionActuationMode=InputMotion  SensePosition=on  SenseVelocity=on  SenseAcceleration=on  SenseTorqueForce=on  SenseLowerLimitTorqueForce=off  SenseUpperLimitTorqueForce=off  LowerLimitSpecify=off  LowerLimitBound=0  LowerLimitBoundUnits=rad  LowerLimitStiffness=1e4  LowerLimitStiffnessUnits=N*m/deg  LowerLimitDamping=10  LowerLimitDampingUnits=N*m/(deg/s)  LowerLimitTransitionRegionWidth=0.1  LowerLimitTransitionRegionWidthUnits=deg  UpperLimitSpecify=off  UpperLimitBound=0  UpperLimitBoundUnits=rad  UpperLimitStiffness=1e4  UpperLimitStiffnessUnits=N*m/deg  UpperLimitDamping=10  UpperLimitDampingUnits=N*m/(deg/s)  UpperLimitTransitionRegionWidth=0.1  UpperLimitTransitionRegionWidthUnits=deg  PositionTargetSpecify=off  PositionTargetPriority=High  PositionTargetValue=0  PositionTargetValueUnits=deg  VelocityTargetSpecify=off  VelocityTargetPriority=High  VelocityTargetValue=0  VelocityTargetValueUnits=deg/s
  Right_Thigh_Joint : sm_lib/Joints/Revolute Joint  JointMode=Normal  SenseConstraintForce=off  SenseConstraintForceX=off  SenseConstraintForceY=off  SenseConstraintForceZ=off  SenseConstraintTorque=off  SenseConstraintTorqueX=off  SenseConstraintTorqueY=off  SenseConstraintTorqueZ=off  SenseTotalForce=off  SenseTotalForceX=off  SenseTotalForceY=off  SenseTotalForceZ=off  SenseTotalTorque=off  SenseTotalTorqueX=off  SenseTotalTorqueY=off  SenseTotalTorqueZ=off  CompositeWrenchDir=FollowerOnBase  CompositeWrenchFrame=BaseFrame  EquilibriumPosition=0  EquilibriumPositionUnits=deg  SpringStiffness=0  SpringStiffnessUnits=N*m/deg  DampingCoefficient=0  DampingCoefficientUnits=m^2*kg/s/rad  TorqueActuationMode=ComputedTorque  MotionActuationMode=InputMotion  SensePosition=on  SenseVelocity=on  SenseAcceleration=on  SenseTorqueForce=on  SenseLowerLimitTorqueForce=off  SenseUpperLimitTorqueForce=off  LowerLimitSpecify=off  LowerLimitBound=0  LowerLimitBoundUnits=rad  LowerLimitStiffness=1e4  LowerLimitStiffnessUnits=N*m/deg  LowerLimitDamping=10  LowerLimitDampingUnits=N*m/(deg/s)  LowerLimitTransitionRegionWidth=0.1  LowerLimitTransitionRegionWidthUnits=deg  UpperLimitSpecify=off  UpperLimitBound=0  UpperLimitBoundUnits=rad  UpperLimitStiffness=1e4  UpperLimitStiffnessUnits=N*m/deg  UpperLimitDamping=10  UpperLimitDampingUnits=N*m/(deg/s)  UpperLimitTransitionRegionWidth=0.1  UpperLimitTransitionRegionWidthUnits=deg  PositionTargetSpecify=off  PositionTargetPriority=High  PositionTargetValue=0  PositionTargetValueUnits=deg  VelocityTargetSpecify=off  VelocityTargetPriority=High  VelocityTargetValue=0  VelocityTargetValueUnits=deg/s
  Right_Thigh_Link : Subsystem
  Simulink-PS Converter{,2,4..9} (8 alike) : nesl_utility/Simulink-PS Converter  PhysicalDomain=network_engine_domain  SubClassName=ps_input  LeftPortType=input  RightPortType=output  PseudoPeriodic=off  Frequencies=[]  NoiseDistribution=none  NoiseParameters=[]  Unit=rad  AffineConversion=off  FilteringAndDerivatives=zero  SimscapeFilterOrder=1  InputFilterTimeConstant=0.001  UdotUserProvided=2
  Solver Configuration1 : nesl_utility/Solver Configuration  PhysicalDomain=network_engine_domain  SubClassName=solver  LeftPortType=input  RightPortType=generic  Tones=[]  Harmonics=[]  SimulateNoise=off  Profile=off  UseLocalSampling=off  EnableSwitchedLinearOptims=on  FrequencyDomain=off  UseCCode=off  RelTol=0.001  AbsTol=1e-06  MinStep=1e-09  ToWorkspace=off  RevertToSquareIcSolve=off  NumHomotopyIterations=100  PhasorMode=off  PhasorModeNumHarmonics=1  DoDC=off  ResidualTolerance=1e-09  UseLocalSolver=off  LocalSolverChoice=NE_BACKWARD_EULER_ADVANCER  LocalSolverSampleTime=0.001  DoFixedCost=off  MaxNonlinIter=3  MaxModeIter=2  LinearAlgebra=auto  EquationFormulation=NE_TIME_EF  DelaysMemoryBudget=1024  AutomaticFiltering=on  FilteringTimeConstant=0.001  PartitionStorageMethod=AS_NEEDED  PartitionMemoryBudget=1024  PartitionMethod=ROBUST
  World1 : sm_lib/Frames and Transforms/World Frame
  left_hip_position : Outport  VectorParamsAs1DForOutWhenUnconnected=off
  left_hip_velocity : Outport  Port=2  VectorParamsAs1DForOutWhenUnconnected=off
  left_hip_acceleration : Outport  Port=3  VectorParamsAs1DForOutWhenUnconnected=off
  left_hip_torque : Outport  Port=4  VectorParamsAs1DForOutWhenUnconnected=off
  left_thigh_position : Outport  Port=5  VectorParamsAs1DForOutWhenUnconnected=off
  left_thigh_velocity : Outport  Port=6  VectorParamsAs1DForOutWhenUnconnected=off
  left_thigh_acceleration : Outport  Port=7  VectorParamsAs1DForOutWhenUnconnected=off
  left_thigh_torque : Outport  Port=8  VectorParamsAs1DForOutWhenUnconnected=off
  left_knee_position : Outport  Port=9  VectorParamsAs1DForOutWhenUnconnected=off
  left_knee_velocity : Outport  Port=10  VectorParamsAs1DForOutWhenUnconnected=off
  left_knee_acceleration : Outport  Port=11  VectorParamsAs1DForOutWhenUnconnected=off
  left_knee_torque : Outport  Port=12  VectorParamsAs1DForOutWhenUnconnected=off
  left_ankle_position : Outport  Port=13  VectorParamsAs1DForOutWhenUnconnected=off
  left_ankle_velocity : Outport  Port=14  VectorParamsAs1DForOutWhenUnconnected=off
  left_ankle_acceleration : Outport  Port=15  VectorParamsAs1DForOutWhenUnconnected=off
  left_ankle_torque : Outport  Port=16  VectorParamsAs1DForOutWhenUnconnected=off
  right_hip_position : Outport  Port=17  VectorParamsAs1DForOutWhenUnconnected=off
  right_hip_velocity : Outport  Port=18  VectorParamsAs1DForOutWhenUnconnected=off
  right_hip_acceleration : Outport  Port=19  VectorParamsAs1DForOutWhenUnconnected=off
  right_hip_torque : Outport  Port=20  VectorParamsAs1DForOutWhenUnconnected=off
  right_thigh_position : Outport  Port=21  VectorParamsAs1DForOutWhenUnconnected=off
  right_thigh_velocity : Outport  Port=22  VectorParamsAs1DForOutWhenUnconnected=off
  right_thigh_acceleration : Outport  Port=23  VectorParamsAs1DForOutWhenUnconnected=off
  right_thigh_torque : Outport  Port=24  VectorParamsAs1DForOutWhenUnconnected=off
  right_knee_position : Outport  Port=25  VectorParamsAs1DForOutWhenUnconnected=off
  right_knee_velocity : Outport  Port=26  VectorParamsAs1DForOutWhenUnconnected=off
  right_knee_acceleration : Outport  Port=27  VectorParamsAs1DForOutWhenUnconnected=off
  right_knee_torque : Outport  Port=28  VectorParamsAs1DForOutWhenUnconnected=off
  right_ankle_position : Outport  Port=29  VectorParamsAs1DForOutWhenUnconnected=off
  right_ankle_velocity : Outport  Port=30  VectorParamsAs1DForOutWhenUnconnected=off
  right_ankle_acceleration : Outport  Port=31  VectorParamsAs1DForOutWhenUnconnected=off
  right_ankle_torque : Outport  Port=32  VectorParamsAs1DForOutWhenUnconnected=off
  wires:
  PS-Simulink Converter36/1 -> Rate Transition57/1
  P_left_ankle/1 -> Rate Transition61/1
  Rate Transition50/1 -> left_knee_torque/1
  Rate Transition53/1 -> left_knee_position/1
  PS-Simulink Converter39/1 -> Rate Transition54/1
  Rate Transition55/1 -> left_ankle_acceleration/1
  Rate Transition57/1 -> left_ankle_position/1
  PS-Simulink Converter37/1 -> Rate Transition56/1
  PS-Simulink Converter27/1 -> Rate Transition42/1
  PS-Simulink Converter38/1 -> Rate Transition55/1
  Rate Transition61/1 -> Simulink-PS Converter9/1
  PS-Simulink Converter30/1 -> Rate Transition47/1
  PS-Simulink Converter31/1 -> Rate Transition46/1
  Rate Transition46/1 -> left_thigh_torque/1
  Rate Transition60/1 -> Simulink-PS Converter8/1
  PS-Simulink Converter28/1 -> Rate Transition49/1
  Rate Transition49/1 -> left_thigh_position/1
  Rate Transition44/1 -> left_hip_velocity/1
  PS-Simulink Converter33/1 -> Rate Transition52/1
  PS-Simulink Converter32/1 -> Rate Transition53/1
  PS-Simulink Converter29/1 -> Rate Transition48/1
  Rate Transition52/1 -> left_knee_velocity/1
  Rate Transition54/1 -> left_ankle_torque/1
  Rate Transition51/1 -> left_knee_acceleration/1
  PS-Simulink Converter35/1 -> Rate Transition50/1
  Rate Transition56/1 -> left_ankle_velocity/1
  Rate Transition42/1 -> left_hip_torque/1
  Rate Transition45/1 -> left_hip_position/1
  Rate Transition59/1 -> Simulink-PS Converter7/1
  Rate Transition43/1 -> left_hip_acceleration/1
  Rate Transition58/1 -> Simulink-PS Converter6/1
  Rate Transition47/1 -> left_thigh_acceleration/1
  PS-Simulink Converter24/1 -> Rate Transition45/1
  P_left_knee/1 -> Rate Transition60/1
  P_left_hip/1 -> Rate Transition58/1
  Rate Transition48/1 -> left_thigh_velocity/1
  P_left_thigh/1 -> Rate Transition59/1
  PS-Simulink Converter25/1 -> Rate Transition44/1
  PS-Simulink Converter26/1 -> Rate Transition43/1
  PS-Simulink Converter34/1 -> Rate Transition51/1
  P_right_knee/1 -> Rate Transition36/1
  Rate Transition16/1 -> right_ankle_torque/1
  P_right_ankle/1 -> Rate Transition37/1
  PS-Simulink Converter15/1 -> Rate Transition14/1
  PS-Simulink Converter14/1 -> Rate Transition15/1
  Rate Transition15/1 -> right_ankle_position/1
  PS-Simulink Converter/1 -> Rate Transition9/1
  PS-Simulink Converter3/1 -> Rate Transition6/1
  PS-Simulink Converter4/1 -> Rate Transition4/1
  PS-Simulink Converter10/1 -> Rate Transition10/1
  Rate Transition6/1 -> right_hip_torque/1
  Rate Transition9/1 -> right_hip_position/1
  Rate Transition2/1 -> right_thigh_acceleration/1
  PS-Simulink Converter12/1 -> Rate Transition13/1
  PS-Simulink Converter1/1 -> Rate Transition8/1
  Rate Transition34/1 -> Simulink-PS Converter2/1
  P_right_hip/1 -> Rate Transition/1
  PS-Simulink Converter7/1 -> Rate Transition1/1
  Rate Transition8/1 -> right_hip_velocity/1
  P_right_thigh/1 -> Rate Transition34/1
  Rate Transition7/1 -> right_hip_acceleration/1
  Rate Transition14/1 -> right_ankle_velocity/1
  Rate Transition37/1 -> Simulink-PS Converter5/1
  Rate Transition36/1 -> Simulink-PS Converter4/1
  Rate Transition5/1 -> right_knee_torque/1
  PS-Simulink Converter8/1 -> Rate Transition12/1
  Rate Transition11/1 -> right_knee_velocity/1
  Rate Transition12/1 -> right_knee_position/1
  Rate Transition1/1 -> right_thigh_torque/1
  Rate Transition/1 -> Simulink-PS Converter/1
  PS-Simulink Converter5/1 -> Rate Transition3/1
  PS-Simulink Converter6/1 -> Rate Transition2/1
  Rate Transition13/1 -> right_ankle_acceleration/1
  PS-Simulink Converter2/1 -> Rate Transition7/1
  Rate Transition4/1 -> right_thigh_position/1
  PS-Simulink Converter11/1 -> Rate Transition5/1
  PS-Simulink Converter9/1 -> Rate Transition11/1
  Rate Transition10/1 -> right_knee_acceleration/1
  PS-Simulink Converter13/1 -> Rate Transition16/1
  Rate Transition3/1 -> right_thigh_velocity/1
  connections:
  Left_Thight_Joint/RConn4 -- PS-Simulink Converter30/LConn1
  Back_Base_Link/RConn2 -- Left_Hip_Joint/LConn1
  Left_Knee_Joint/RConn4 -- PS-Simulink Converter34/LConn1
  Left_Hip_Joint/RConn1 -- Left_Hip_Link/LConn1
  Simulink-PS Converter8/RConn1 -- Left_Knee_Joint/LConn2
  PS-Simulink Converter27/LConn1 -- Left_Hip_Joint/RConn5
  PS-Simulink Converter35/LConn1 -- Left_Knee_Joint/RConn5
  Left_Knee_Joint/RConn1 -- Left_Calf_Link/LConn1
  PS-Simulink Converter32/LConn1 -- Left_Knee_Joint/RConn2
  PS-Simulink Converter39/LConn1 -- Left_Ankle_Joint/RConn5
  Left_Thigh_Link/LConn1 -- Left_Thight_Joint/RConn1
  Simulink-PS Converter7/RConn1 -- Left_Thight_Joint/LConn2
  Simulink-PS Converter6/RConn1 -- Left_Hip_Joint/LConn2
  Left_Ankle_Joint/RConn4 -- PS-Simulink Converter38/LConn1
  PS-Simulink Converter28/LConn1 -- Left_Thight_Joint/RConn2
  Left_Ankle_Joint/LConn1 -- Left_Calf_Link/RConn1
  Left_Knee_Joint/LConn1 -- Left_Thigh_Link/RConn1
  PS-Simulink Converter25/LConn1 -- Left_Hip_Joint/RConn3
  PS-Simulink Converter36/LConn1 -- Left_Ankle_Joint/RConn2
  PS-Simulink Converter26/LConn1 -- Left_Hip_Joint/RConn4
  PS-Simulink Converter24/LConn1 -- Left_Hip_Joint/RConn2
  PS-Simulink Converter31/LConn1 -- Left_Thight_Joint/RConn5
  Left_Hip_Link/RConn1 -- Left_Thight_Joint/LConn1
  Left_Ankle_Joint/RConn1 -- Left_Ankle_Link/LConn1
  Left_Knee_Joint/RConn3 -- PS-Simulink Converter33/LConn1
  Simulink-PS Converter9/RConn1 -- Left_Ankle_Joint/LConn2
  Left_Thight_Joint/RConn3 -- PS-Simulink Converter29/LConn1
  Left_Ankle_Joint/RConn3 -- PS-Simulink Converter37/LConn1
  MechanismConfiguration/RConn1 -- Back_Base_Link/LConn1 -- World1/RConn1 -- Solver Configuration1/RConn1
  Back_Base_Link/RConn1 -- Right_Hip_Joint/LConn1
  PS-Simulink Converter4/LConn1 -- Right_Thigh_Joint/RConn2
  PS-Simulink Converter13/LConn1 -- Right_Ankle_Joint/RConn5
  Right_Knee_Joint/LConn2 -- Simulink-PS Converter4/RConn1
  PS-Simulink Converter7/LConn1 -- Right_Thigh_Joint/RConn5
  PS-Simulink Converter15/LConn1 -- Right_Ankle_Joint/RConn3
  Right_Thigh_Joint/RConn1 -- Right_Thigh_Link/LConn1
  PS-Simulink Converter2/LConn1 -- Right_Hip_Joint/RConn4
  Right_Knee_Joint/LConn1 -- Right_Thigh_Link/RConn1
  PS-Simulink Converter11/LConn1 -- Right_Knee_Joint/RConn5
  Right_Knee_Joint/RConn1 -- Right_Calf_Link/LConn1
  Simulink-PS Converter/RConn1 -- Right_Hip_Joint/LConn2
  Right_Ankle_Joint/LConn1 -- Right_Calf_Link/RConn1
  PS-Simulink Converter14/LConn1 -- Right_Ankle_Joint/RConn2
  PS-Simulink Converter1/LConn1 -- Right_Hip_Joint/RConn3
  Right_Ankle_Joint/RConn1 -- Right_Ankle_Link/LConn1
  PS-Simulink Converter3/LConn1 -- Right_Hip_Joint/RConn5
  Right_Hip_Joint/RConn1 -- Right_Hip_Link/LConn1
  Right_Hip_Link/RConn1 -- Right_Thigh_Joint/LConn1
  PS-Simulink Converter12/LConn1 -- Right_Ankle_Joint/RConn4
  PS-Simulink Converter10/LConn1 -- Right_Knee_Joint/RConn4
  Simulink-PS Converter5/RConn1 -- Right_Ankle_Joint/LConn2
  PS-Simulink Converter9/LConn1 -- Right_Knee_Joint/RConn3
  PS-Simulink Converter6/LConn1 -- Right_Thigh_Joint/RConn4
  PS-Simulink Converter8/LConn1 -- Right_Knee_Joint/RConn2
  PS-Simulink Converter5/LConn1 -- Right_Thigh_Joint/RConn3
  Right_Thigh_Joint/LConn2 -- Simulink-PS Converter2/RConn1
  PS-Simulink Converter/LConn1 -- Right_Hip_Joint/RConn2

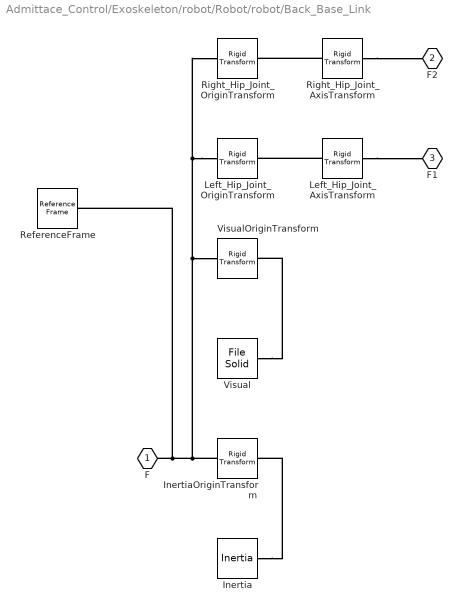
== system Admittace_Control/Exoskeleton/robot/Robot/robot/Back_Base_Link ==
  Inertia : sm_lib/Body Elements/Inertia  InertiaType=Custom  Mass=7.1666344893724  MassUnits=kg  CenterOfMass=[0, 0, 0]  CenterOfMassUnits=m  MomentsOfInertia=[0.287991764742564, 0.218183102338654, 0.12372998211452]  MomentsOfInertiaUnits=kg*m^2  ProductsOfInertia=[-5.72291606644722e-09, 0.00975876307734881, 4.03119244398634e-09]  ProductsOfInertiaUnits=kg*m^2  GraphicType=None  MarkerShape=Inertia  MarkerSize=20  GraphicVisPropType=SimpleVisualProperties  GraphicDiffuseColor=[0.5 0.5 0.5]  GraphicSpecularColor=[0.5 0.5 0.5 1.0]  GraphicAmbientColor=[0.15 0.15 0.15 1.0]  GraphicEmissiveColor=[0.0 0.0 0.0 1.0]  GraphicShininess=75  GraphicOpacity=1.0
  InertiaOriginTransform : sm_lib/Frames and Transforms/Rigid Transform  TranslationMethod=Cartesian  TranslationStandardOffset=0  TranslationLengthUnit=m  TranslationStandardAxis=+Z  TranslationCartesianOffset=[0.102999774541297, 1.05565171604205e-08, -0.01817224156931]  TranslationROffset=0  TranslationROffsetUnits=m  TranslationZOffset=0  TranslationZOffsetUnits=m  TranslationThetaOffset=0  TranslationThetaOffsetUnits=deg  RotationMethod=RotationSequence  RotationAngleUnits=deg  RotationStandardAxis=+Z  RotationAngle=0.0  RotationArbitraryAxis=[0 0 1]  FollAlignAxisA=+X  BaseAlignAxisA=+Y  FollAlignAxisB=+Y  BaseAlignAxisB=+Z  RotationSequenceAxes=BaseAxes  RotationSequence=XYZ  RotationSequenceAngles=[0, 0, 0]  RotationSequenceAnglesUnits=rad  RotationMatrix=[1 0 0; 0 1 0; 0 0 1]
  Left_Hip_Joint_AxisTransform : sm_lib/Frames and Transforms/Rigid Transform  TranslationMethod=Cartesian  TranslationStandardOffset=0  TranslationLengthUnit=m  TranslationStandardAxis=+Z  TranslationCartesianOffset=[0, 0, 0]  TranslationROffset=0  TranslationROffsetUnits=m  TranslationZOffset=0  TranslationZOffsetUnits=m  TranslationThetaOffset=0  TranslationThetaOffsetUnits=deg  RotationMethod=ArbitraryAxis  RotationAngleUnits=rad  RotationStandardAxis=+Z  RotationAngle=3.141592653589793  RotationArbitraryAxis=[1, 0, 0]  FollAlignAxisA=+X  BaseAlignAxisA=+Y  FollAlignAxisB=+Y  BaseAlignAxisB=+Z  RotationSequenceAxes=FollowerAxes  RotationSequence=XYX  RotationSequenceAngles=[0 0 0]  RotationSequenceAnglesUnits=deg  RotationMatrix=[1 0 0; 0 1 0; 0 0 1]
  Left_Hip_Joint_OriginTransform : sm_lib/Frames and Transforms/Rigid Transform  TranslationMethod=Cartesian  TranslationStandardOffset=0  TranslationLengthUnit=m  TranslationStandardAxis=+Z  TranslationCartesianOffset=[0.2243, 0.208, -0.283]  TranslationROffset=0  TranslationROffsetUnits=m  TranslationZOffset=0  TranslationZOffsetUnits=m  TranslationThetaOffset=0  TranslationThetaOffsetUnits=deg  RotationMethod=RotationSequence  RotationAngleUnits=deg  RotationStandardAxis=+Z  RotationAngle=0.0  RotationArbitraryAxis=[0 0 1]  FollAlignAxisA=+X  BaseAlignAxisA=+Y  FollAlignAxisB=+Y  BaseAlignAxisB=+Z  RotationSequenceAxes=BaseAxes  RotationSequence=XYZ  RotationSequenceAngles=[0, 0, 0]  RotationSequenceAnglesUnits=rad  RotationMatrix=[1 0 0; 0 1 0; 0 0 1]
  ReferenceFrame : sm_lib/Frames and Transforms/Reference Frame
  Right_Hip_Joint_AxisTransform : sm_lib/Frames and Transforms/Rigid Transform  TranslationMethod=Cartesian  TranslationStandardOffset=0  TranslationLengthUnit=m  TranslationStandardAxis=+Z  TranslationCartesianOffset=[0, 0, 0]  TranslationROffset=0  TranslationROffsetUnits=m  TranslationZOffset=0  TranslationZOffsetUnits=m  TranslationThetaOffset=0  TranslationThetaOffsetUnits=deg  RotationMethod=ArbitraryAxis  RotationAngleUnits=rad  RotationStandardAxis=+Z  RotationAngle=0  RotationArbitraryAxis=[1, 0, 0]  FollAlignAxisA=+X  BaseAlignAxisA=+Y  FollAlignAxisB=+Y  BaseAlignAxisB=+Z  RotationSequenceAxes=FollowerAxes  RotationSequence=XYX  RotationSequenceAngles=[0 0 0]  RotationSequenceAnglesUnits=deg  RotationMatrix=[1 0 0; 0 1 0; 0 0 1]
  Right_Hip_Joint_OriginTransform : sm_lib/Frames and Transforms/Rigid Transform  TranslationMethod=Cartesian  TranslationStandardOffset=0  TranslationLengthUnit=m  TranslationStandardAxis=+Z  TranslationCartesianOffset=[0.2243, -0.208, -0.283]  TranslationROffset=0  TranslationROffsetUnits=m  TranslationZOffset=0  TranslationZOffsetUnits=m  TranslationThetaOffset=0  TranslationThetaOffsetUnits=deg  RotationMethod=RotationSequence  RotationAngleUnits=deg  RotationStandardAxis=+Z  RotationAngle=0.0  RotationArbitraryAxis=[0 0 1]  FollAlignAxisA=+X  BaseAlignAxisA=+Y  FollAlignAxisB=+Y  BaseAlignAxisB=+Z  RotationSequenceAxes=BaseAxes  RotationSequence=XYZ  RotationSequenceAngles=[0, 0, 0]  RotationSequenceAnglesUnits=rad  RotationMatrix=[1 0 0; 0 1 0; 0 0 1]
  Visual : sm_lib/Body Elements/File Solid  ExtGeomFileName=C:\Users\河明山\Desktop\毕业设计\下肢\meshes\Back_Base_Link.STL  UnitType=Custom  ExtGeomFileUnits=m  StepReaderType=HEX  ExportConvexHullGeometry=off  InertiaType=Custom  Mass=0  MassUnits=kg  CenterOfMass=[0, 0, 0]  CenterOfMassUnits=m  MomentsOfInertia=[0, 0, 0]  MomentsOfInertiaUnits=kg*m^2  ProductsOfInertia=[0, 0, 0]  ProductsOfInertiaUnits=kg*m^2  BasedOnType=DensityFromFile  Density=1000  DensityUnits=kg/m^3  DoExposeReferenceFrame=on  SerializedFrames=<Frames/>  GraphicType=FromGeometry  MarkerShape=Sphere  MarkerSize=10  GraphicVisPropType=SimpleVisualProperties  GraphicDiffuseColor=[0.898039215686275, 0.917647058823529, 0.929411764705882]  GraphicSpecularColor=[0.5 0.5 0.5 1.0]  GraphicAmbientColor=[0.15 0.15 0.15 1.0]  GraphicEmissiveColor=[0.0 0.0 0.0 1.0]  GraphicShininess=75  GraphicOpacity=1
  VisualOriginTransform : sm_lib/Frames and Transforms/Rigid Transform  TranslationMethod=Cartesian  TranslationStandardOffset=0  TranslationLengthUnit=m  TranslationStandardAxis=+Z  TranslationCartesianOffset=[0, 0, 0]  TranslationROffset=0  TranslationROffsetUnits=m  TranslationZOffset=0  TranslationZOffsetUnits=m  TranslationThetaOffset=0  TranslationThetaOffsetUnits=deg  RotationMethod=RotationSequence  RotationAngleUnits=deg  RotationStandardAxis=+Z  RotationAngle=0.0  RotationArbitraryAxis=[0 0 1]  FollAlignAxisA=+X  BaseAlignAxisA=+Y  FollAlignAxisB=+Y  BaseAlignAxisB=+Z  RotationSequenceAxes=BaseAxes  RotationSequence=XYZ  RotationSequenceAngles=[0, 0, 0]  RotationSequenceAnglesUnits=rad  RotationMatrix=[1 0 0; 0 1 0; 0 0 1]
  F : PMIOPort  Side=Left
  F2 : PMIOPort  Port=2  Side=Right
  F1 : PMIOPort  Port=3  Side=Right
  connections:
  Inertia/RConn1 -- InertiaOriginTransform/RConn1
  Left_Hip_Joint_AxisTransform/RConn1 -- F1/RConn1
  Left_Hip_Joint_AxisTransform/LConn1 -- Left_Hip_Joint_OriginTransform/RConn1
  Left_Hip_Joint_OriginTransform/LConn1 -- InertiaOriginTransform/LConn1 -- ReferenceFrame/RConn1 -- F/RConn1 -- VisualOriginTransform/LConn1 -- Right_Hip_Joint_OriginTransform/LConn1
  Right_Hip_Joint_AxisTransform/RConn1 -- F2/RConn1
  Right_Hip_Joint_AxisTransform/LConn1 -- Right_Hip_Joint_OriginTransform/RConn1
  Visual/RConn1 -- VisualOriginTransform/RConn1
